simulink model "u2w"  (R2019b)
settings: Solver=FixedStepAuto  StartTime=0.0  StopTime=10.0  FixedStep=0.1  RelTol=1e-3
undefined symbols (not defined in the file): Rl, Rr, W
settings Model: Creator=r720r  LastModifiedBy=r720r

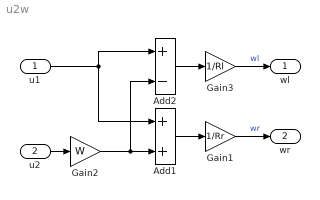
== system u2w ==
  u1 : Inport  OutDataTypeStr=double  PortDimensions=1
  u2 : Inport  Port=2  OutDataTypeStr=double  PortDimensions=1
  Add1 : Sum
  Add2 : Sum  Inputs=+-
  Gain1 : Gain  Gain=1/Rr
  Gain2 : Gain  Gain=W
  Gain3 : Gain  Gain=1/Rl
  wl : Outport  OutDataTypeStr=double  PortDimensions=1
  wr : Outport  Port=2  OutDataTypeStr=double  PortDimensions=1
  wires:
  Gain3/1 -> wl/1  "wl"
  u1/1 -> Add1/1, Add2/1
  u2/1 -> Gain2/1
  Add2/1 -> Gain3/1
  Gain2/1 -> Add1/2, Add2/2
  Gain1/1 -> wr/1  "wr"
  Add1/1 -> Gain1/1
